simulink model "lab2_FW"  (R2023a)
settings: Solver=VariableStepAuto  StartTime=0.0  StopTime=0  RelTol=1e-3
undefined symbols (not defined in the file or in its folder): Rec, SDTV
libraries: visionsinks x2, visionsources x1, visionconversions x1
settings Model: Creator=alexa  LastModifiedBy=alexa
settings DebuggingCC: UnconnectedInputMsg=warning  UnconnectedOutputMsg=warning  UnconnectedLineMsg=warning
settings ModelReferenceCC: EnableRefExpFcnMdlSchedulingChecks=on
settings RTWCC: DLArmComputeVersion=19.05

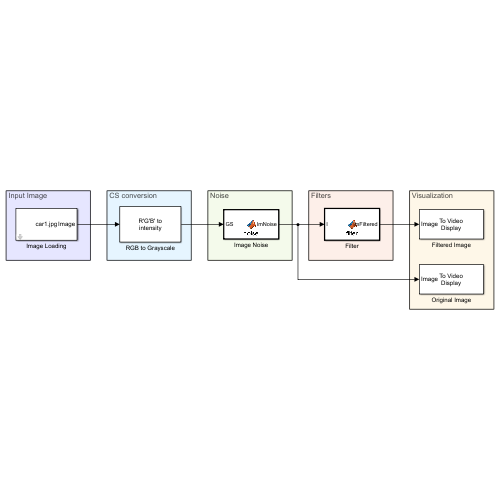
[thumbnail: Simulink's stored preview of the top-level diagram]
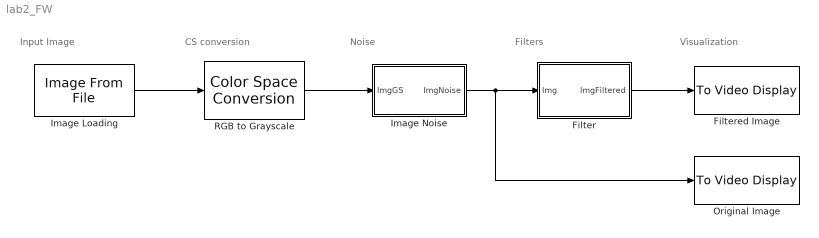
== system lab2_FW ==
  note: Input Image
  note: CS conversion
  note: Noise
  note: Filters
  note: Visualization
  Filter : MATLAB Function  TreatAsAtomicUnit=on
  Filtered Image : visionsinks/To Video Display  windowSizeMode=Normal  openAtMdlStart=on  fullScreen=off  videoWindowX=815  videoWindowY=-1455  saveWindowSize=off  videoWindowWidth=854  videoWindowHeight=872  inputColorFormat=RGB  inputType=Obsolete  imagePorts=One multidimensional signal  OutputDevice=On-screen video monitor  dataOrg=Column-major  isWindowOpen=on
  Image Loading : visionsources/Image From File  Tag=vipblks_nd  FileName=car1.jpg  Ts=0.01  imagePorts=One multidimensional signal  OutPortLabels=R|G|B  ImageDataType=double  sdImageDataType=uint(8)  Signed=on  WordLength=16  FractionLengthMode=User-defined  FractionLength=15
  Image Noise : MATLAB Function  TreatAsAtomicUnit=on
  Original Image : visionsinks/To Video Display  windowSizeMode=Normal  openAtMdlStart=on  fullScreen=off  videoWindowX=1713  videoWindowY=-1322  saveWindowSize=off  videoWindowWidth=854  videoWindowHeight=872  inputColorFormat=RGB  inputType=Obsolete  imagePorts=One multidimensional signal  OutputDevice=On-screen video monitor  dataOrg=Column-major  isWindowOpen=on
  RGB to Grayscale : visionconversions/Color Space  Conversion  conversion=Obsolete  conversionActive=R'G'B' to intensity  wp_str=D65  rec=Rec. 601 (SDTV)  sys=1125/60/2:1  imagePorts=One multidimensional signal
  wires:
  Image Loading/1 -> RGB to Grayscale/1
  RGB to Grayscale/1 -> Image Noise/1(ImgGS)
  Image Noise/1(ImgNoise) -> Original Image/1, Filter/1(Img)
  Filter/1(ImgFiltered) -> Filtered Image/1

== matlab function lab2_FW/Filter ==
  data: Img input double; ImgFiltered output double
function ImgFiltered = filter(Img)
% Use the code below to include the function you want to use
% coder.extrinsic('function');

% Call the function you want to use and call its output "outvar"
outvar = Img;

% Function output (do not change!)
ImgFiltered = coder.nullcopy(zeros(size(Img)));
ImgFiltered = double(outvar);
end

== matlab function lab2_FW/Image Noise ==
  data: ImgGS input; ImgNoise output
function ImgNoise = noise(ImgGS)
% Use the code below to include the function you want to use
% coder.extrinsic('function');

% Call the function you want to use and call its output "outvar"
outvar = ImgGS;

% Function output (do not change!)
ImgNoise = coder.nullcopy(zeros(size(ImgGS)));
ImgNoise = double(outvar);
end
